simulink model "robot"  (R2025b)
settings: Solver=VariableStepAuto  StartTime=0.0  StopTime=10.0  MaxStep=0.2  RelTol=1e-3
PostLoadFcn:
  | rigid_body = importrobot('urdf\iiwa7\iiwa7.urdf');
  | rigid_body.DataFormat = 'column';
  | rigid_body.Gravity = [0 0 -9.81];
libraries: aerolibanimutils x1, robotmaniplib x1
settings Model: Creator=Junch  LastModifiedBy=Junch

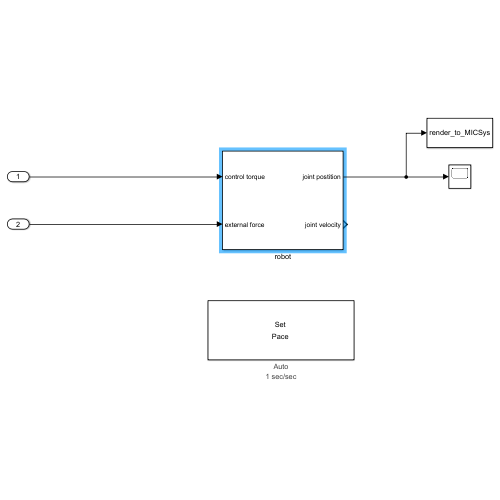
[thumbnail: Simulink's stored preview of the top-level diagram]
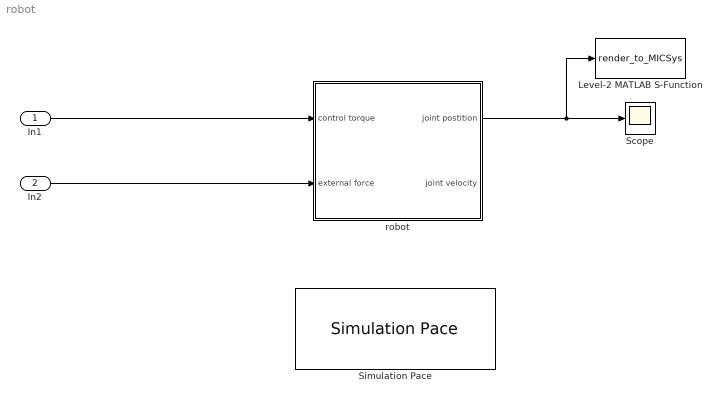
== system robot ==
  In1 : Inport
  In2 : Inport  Port=2
  Level-2 MATLAB S-Function : M-S-Function  FunctionName=render_to_MICSys
  Scope : Scope
      settings: ActiveDisplayYMinimum=-1  ActiveDisplayYMaximum=1
  Simulation Pace : aerolibanimutils/Simulation Pace  SimulationPace=1  SleepMode=Auto  OutputPaceError=off  SampleTime=1/30
  robot : Subsystem
  wires:
  In1/1 -> robot/1(control torque)
  In2/1 -> robot/2(external force)
  robot/1(joint postition) -> Level-2 MATLAB S-Function/1, Scope/1

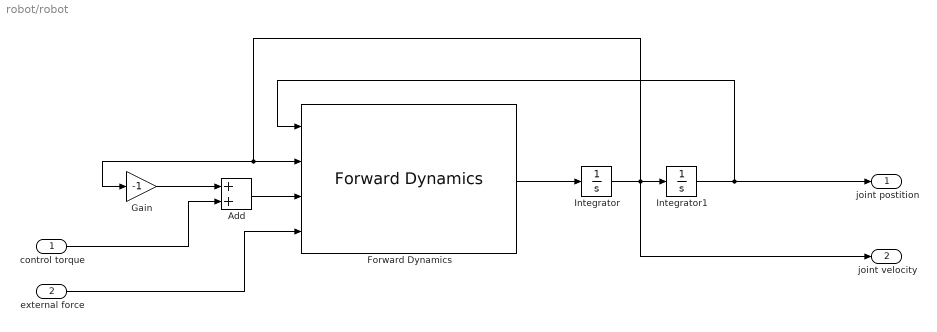
== system robot/robot ==
  control torque : Inport
  external force : Inport  Port=2
  Add : Sum
  Forward Dynamics : robotmaniplib/Forward Dynamics  RigidBodyTree=rigid_body  SimulateUsing=Interpreted execution
  Gain : Gain  Gain=-1
  Integrator : Integrator
  Integrator1 : Integrator
  joint postition : Outport
  joint velocity : Outport  Port=2
  wires:
  external force/1 -> Forward Dynamics/4
  Integrator/1 -> joint velocity/1, Gain/1, Forward Dynamics/2, Integrator1/1
  Integrator1/1 -> joint postition/1, Forward Dynamics/1
  Gain/1 -> Add/1
  Forward Dynamics/1 -> Integrator/1
  Add/1 -> Forward Dynamics/3
  control torque/1 -> Add/2
